simulink library "hyblib"  (Simulink 7.3)
settings: Solver=ode45  SolverMode=SingleTasking  StartTime=0.0  StopTime=10.0  RelTol=1e-3
undefined symbols (not defined in the file or in its folder): nu
settings Model: Creator=Alberto Bemporad  LastModifiedBy=bemporad

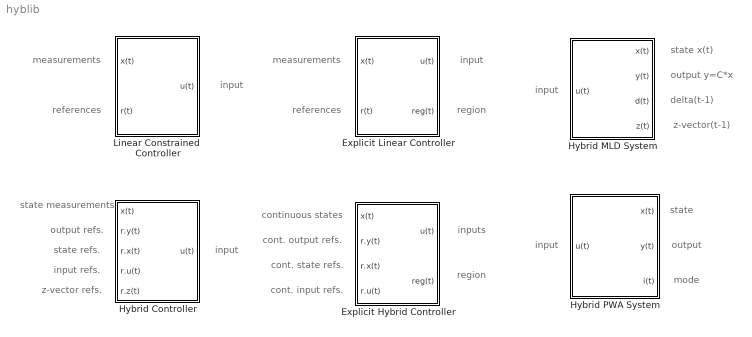
== system hyblib ==
  note: input
  note: references
  note: measurements
  note: input
  note: references
  note: measurements
  note: region
  note: input
  note: state refs.
  note: state
      | measurements
  note: input refs.
  note: z-vector refs.
  note: input
  note: state x(t)
  note: delta(t-1)
  note: z-vector(t-1)
  note: input
  note: mode
  note: inputs
  note: region
  note: cont. state refs.
  note: continuous states
  note: cont. input refs.
  note: output refs.
  note: output y=C*x
  note: output
  note: state
  note: cont. output refs.
  Explicit Hybrid Controller : Subsystem  InitFcn=nu=expsfun_init;  mask(Explicit constrained control){C=, compile=on}
      mask prompts: C "Controller"; compile "Generate MEX file"
      mask Help: The controller is based on a valid @EXPCON object based on a hybrid MLD or PWA model.
      mask Display: image(double(imread('expcon2.jpg'))/255);
  Explicit Linear Controller : Subsystem  InitFcn=nu=expsfun_init;  mask(Explicit constrained control){C=, xhat0=[], u1=[], compile=on}
      mask prompts: C "Controller"; xhat0 "Initial state estimate (output-feedback only)"; u1 "Previous input (reference-tracking only)"; compile "Generate MEX file"
      mask Help:
      | The controller is based on a valid @EXPCON object based on a linear constrained model.
      | The controller can be of two kinds:
      | 1) output feedback, which includes a state observer, and can be used for reference tracking;
      | 2) state feedback for regulating the states of the system to the origin.
      mask Display: image(double(imread('expcon1.jpg'))/255);
  Hybrid Controller : Subsystem  mask(Control of hybrid systems based on MIP){C=, S=0, tilim=0}
      mask prompts: C "Controller"; S "MLD model"; tilim "Time limit (CPLEX and GLPK only. 0 or Inf = unbounded)"
      mask Help:
      | Controller based on on-line mixed-integer linear optimization for constrained hybrid systems.
      | The controller is based on a valid @HYBCON object.
      mask Display: image(double(imread('hybcon1.jpg'))/255);
  Hybrid MLD System : Subsystem  mask(Hybrid MLD dynamics (open-loop)){S=, x0init=}
      mask prompts: S "MLD model"; x0init "Initial state"
      mask Help: Open loop mixed logical dynamical (MLD) system
      mask Display: image(double(imread('hybmld1.jpg'))/255);
  Hybrid PWA System : Subsystem  mask(Hybrid PWA dynamics (open-loop)){P=, x0init=}
      mask prompts: P "PWA model"; x0init "Initial state"
      mask Help: Hybrid piecewise affine (PWA) dynamics
      mask Display: image(double(imread('hybpwa1.jpg'))/255);
  Linear Constrained  Controller : Subsystem  mask(Constrained control of linear systems (QP)){C=, xhat0=[], u1=[]}
      mask prompts: C "Controller"; xhat0 "Initial state (output-feedback only)"; u1 "Previous Input (reference tracking only)"
      mask Help:
      | Controller based on on-line quadratic optimization for constrained linear systems.
      | The controller is based on a valid @LINCON object.
      mask Display: image(double(imread('lincon1.jpg'))/255);

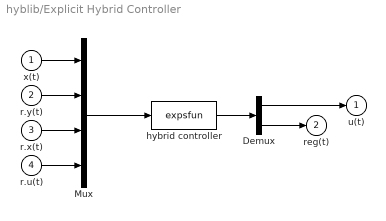
== system hyblib/Explicit Hybrid Controller ==
  x(t) : Inport  OutDataType=sfix(16)  OutScaling=2^0
  r.y(t) : Inport  Port=2  OutDataType=sfix(16)  OutScaling=2^0
  r.x(t) : Inport  Port=3  OutDataType=sfix(16)  OutScaling=2^0
  r.u(t) : Inport  Port=4  OutDataType=sfix(16)  OutScaling=2^0
  Demux : Demux  Outputs=[nu 1]
  Mux : Mux  Inputs=[-1 -1 -1 -1]
  hybrid controller : S-Function  FunctionName=expsfun  EnableBusSupport=off
  u(t) : Outport  InitialOutput=0
  reg(t) : Outport  Port=2  InitialOutput=0
  wires:
  Demux/2 -> reg(t)/1
  Demux/1 -> u(t)/1
  hybrid controller/1 -> Demux/1
  Mux/1 -> hybrid controller/1
  x(t)/1 -> Mux/1
  r.y(t)/1 -> Mux/2
  r.x(t)/1 -> Mux/3
  r.u(t)/1 -> Mux/4

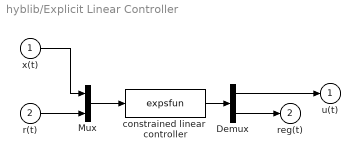
== system hyblib/Explicit Linear Controller ==
  x(t) : Inport  OutDataType=sfix(16)  OutScaling=2^0
  r(t) : Inport  Port=2  OutDataType=sfix(16)  OutScaling=2^0
  Demux : Demux  Outputs=[nu 1]
  Mux : Mux  Inputs=2
  constrained linear  controller : S-Function  FunctionName=expsfun  EnableBusSupport=off
  u(t) : Outport  InitialOutput=0
  reg(t) : Outport  Port=2  InitialOutput=0
  wires:
  Mux/1 -> constrained linear  controller/1
  r(t)/1 -> Mux/2
  x(t)/1 -> Mux/1
  constrained linear  controller/1 -> Demux/1
  Demux/1 -> u(t)/1
  Demux/2 -> reg(t)/1

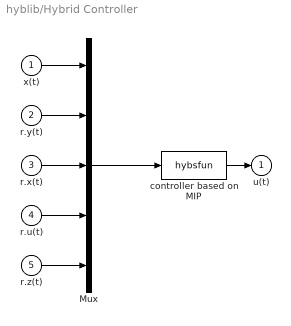
== system hyblib/Hybrid Controller ==
  x(t) : Inport  OutDataType=sfix(16)  OutScaling=2^0
  r.y(t) : Inport  Port=2  OutDataType=sfix(16)  OutScaling=2^0
  r.x(t) : Inport  Port=3  OutDataType=sfix(16)  OutScaling=2^0
  r.u(t) : Inport  Port=4  OutDataType=sfix(16)  OutScaling=2^0
  r.z(t) : Inport  Port=5  OutDataType=sfix(16)  OutScaling=2^0
  Mux : Mux  Inputs=[-1 -1 -1 -1 -1]
  controller based on MIP : S-Function  FunctionName=hybsfun  Parameters=C,S,tilim  EnableBusSupport=off
  u(t) : Outport  InitialOutput=0
  wires:
  x(t)/1 -> Mux/1
  controller based on MIP/1 -> u(t)/1
  r.y(t)/1 -> Mux/2
  r.x(t)/1 -> Mux/3
  r.u(t)/1 -> Mux/4
  r.z(t)/1 -> Mux/5
  Mux/1 -> controller based on MIP/1

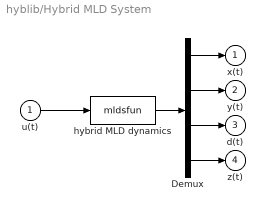
== system hyblib/Hybrid MLD System ==
  u(t) : Inport  OutDataType=sfix(16)  OutScaling=2^0
  Demux : Demux  Outputs=[S.nx+(S.nx==0), S.ny+(S.ny==0), S.nd+(S.nd==0), S.nz+(S.nz==0)]
  hybrid MLD dynamics : S-Function  FunctionName=mldsfun  Parameters=S,x0init  EnableBusSupport=off
  x(t) : Outport  InitialOutput=0
  y(t) : Outport  Port=2  InitialOutput=0
  d(t) : Outport  Port=3  InitialOutput=0
  z(t) : Outport  Port=4  InitialOutput=0
  wires:
  u(t)/1 -> hybrid MLD dynamics/1
  hybrid MLD dynamics/1 -> Demux/1
  Demux/1 -> x(t)/1
  Demux/2 -> y(t)/1
  Demux/3 -> d(t)/1
  Demux/4 -> z(t)/1

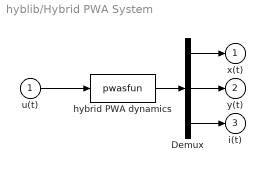
== system hyblib/Hybrid PWA System ==
  u(t) : Inport  OutDataType=sfix(16)  OutScaling=2^0
  Demux : Demux  Outputs=[P.nx+(P.nx==0),P.ny+(P.ny==0),1]
  hybrid PWA dynamics : S-Function  FunctionName=pwasfun  Parameters=P,x0init  EnableBusSupport=off
  x(t) : Outport  InitialOutput=0
  y(t) : Outport  Port=2  InitialOutput=0
  i(t) : Outport  Port=3  InitialOutput=0
  wires:
  hybrid PWA dynamics/1 -> Demux/1
  u(t)/1 -> hybrid PWA dynamics/1
  Demux/3 -> i(t)/1
  Demux/2 -> y(t)/1
  Demux/1 -> x(t)/1

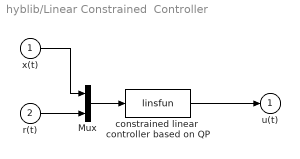
== system hyblib/Linear Constrained  Controller ==
  x(t) : Inport  OutDataType=sfix(16)  OutScaling=2^0
  r(t) : Inport  Port=2  OutDataType=sfix(16)  OutScaling=2^0
  Mux : Mux  Inputs=2
  constrained linear  controller based on QP : S-Function  FunctionName=linsfun  Parameters=C,[],u1  EnableBusSupport=off
  u(t) : Outport  InitialOutput=0
  wires:
  constrained linear  controller based on QP/1 -> u(t)/1
  x(t)/1 -> Mux/1
  r(t)/1 -> Mux/2
  Mux/1 -> constrained linear  controller based on QP/1
